simulink model "testYarpSendBML"  (R2014a)
settings: Solver=FixedStepDiscrete  StartTime=0.0  StopTime=10  FixedStep=0.002  RelTol=1e-3
model workspace (MAT data in the model file):
  gtest = 0
settings Model: Creator=Ulysses  LastModifiedBy=Ulysses

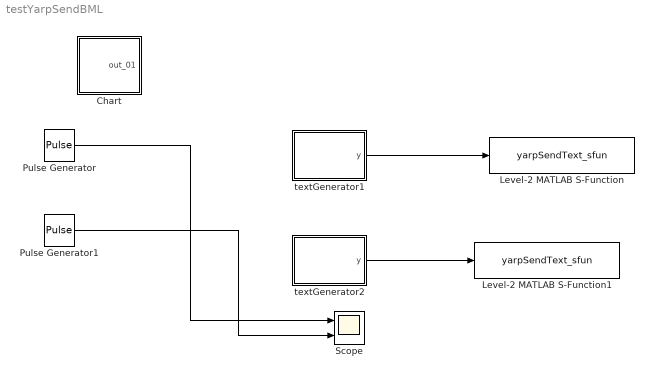
== system testYarpSendBML ==
  Chart : Stateflow chart  TreatAsAtomicUnit=on
  Level-2 MATLAB S-Function : M-S-Function  FunctionName=yarpSendText_sfun  Parameters='/sim/out/bml', '/rr'
  Level-2 MATLAB S-Function1 : M-S-Function  FunctionName=yarpSendText_sfun  Parameters='/sim/out/smb', '/rs'
  Pulse Generator : DiscretePulseGenerator  PulseType=Time based  PulseWidth=5
  Pulse Generator1 : DiscretePulseGenerator  PulseType=Time based  Amplitude=2  PulseWidth=50
  Scope : Scope  NumInputPorts=2
      settings: YMin=-5~-5  YMax=5~5
  textGenerator1 : MATLAB Function  TreatAsAtomicUnit=on
  textGenerator2 : MATLAB Function  TreatAsAtomicUnit=on
  wires:
  Pulse Generator/1 -> Scope/1
  Pulse Generator1/1 -> Scope/2
  textGenerator1/1(y) -> Level-2 MATLAB S-Function/1
  textGenerator2/1(y) -> Level-2 MATLAB S-Function1/1

== matlab function testYarpSendBML/textGenerator1 ==
  data: y output
function y = fcn()
y = encStr2Arr('test string 2');

== matlab function testYarpSendBML/textGenerator2 ==
  data: y output
function y = fcn()
y = encStr2Arr('test string');

== stateflow chart testYarpSendBML/Chart ==
  state state02
    %entry: disp('state02')
    entry: out_01=1
  state state01
    %entry: disp('state01');
  (default) -> state01
  state01 -> state02 : after(2,sec)
  state02 -> state01 : after(2,sec)
  data: out_01 output
